simulink model "relative_distance_tracking4"  (R2018b)
settings: Solver=FixedStepAuto  StartTime=0.0  StopTime=15  FixedStep=dt  RelTol=1e-3
values from neighbouring files (symbols this model uses):
  C = [0 1]    [relative_distance_design4.m]
  CA = C*A    [relative_distance_design4.m]
  d0_ego = 0    [relative_distance_design4.m]
  d0_other = d0_ego + safe_dist0    (= 98.5)    [relative_distance_design4.m]
  fc = 0.5    [relative_distance_design4.m]
  fps2mph = 1/mph2fps    (= 0.680272108844)    [relative_distance_design4.m]
  g = 32.2    [relative_distance_design4.m]    (also in run_decel.m)
  invCB = inv(C*B)    [relative_distance_design4.m]
  Ka = 8    [relative_distance_design4.m]
  Kd = 0.25    [relative_distance_design4.m]
  Kdi = w_des^2    (= 4)    [relative_distance_design4.m]
  Kdp = 2*z_des*w_des    (= 4)    [relative_distance_design4.m]
  Kv = 2    [relative_distance_design4.m]
  max_accel = 0.6*g    (= 19.32)    [relative_distance_design4.m]
  min_accel = -1.0*g    (= -32.2)    [relative_distance_design4.m]
  mph2fps = 1.47    [relative_distance_design4.m]
  safe_dist0 = d0 + slope*(v0_ego*fps2mph)^2 + safe_dist0_margin    (= 98.5)    [relative_distance_design4.m]
  safe_dist_out = d0 + slope*v_in.^2 + safe_dist0_margin    [relative_distance_design4.m]
  v0_ego = 70*mph2fps    (= 102.9)    [relative_distance_design4.m]
  v0_other = v0_ego    (= 102.9)    [relative_distance_design4.m]
  v_in = (0:0.1:100)    [relative_distance_design4.m]
  v_other = v0_other + del_v0    (= 0)    [relative_distance_design4.m]
  wa_ego = 4    [relative_distance_design4.m]
settings Model: Creator=suvo.ganguli  LastModifiedBy=suvo.ganguli

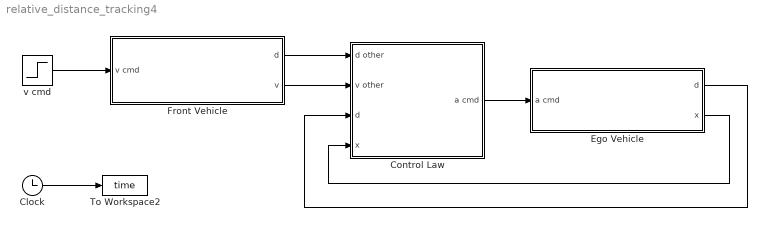
== system relative_distance_tracking4 ==
  Clock : Clock
  Control Law : Subsystem
  Ego Vehicle : Subsystem
  Front Vehicle : Subsystem
  To Workspace2 : ToWorkspace  VariableName=time  SampleTime=-1
  "v cmd " : Step  Before=v0_other  After=v_other  SampleTime=0
  wires:
  Clock/1 -> To Workspace2/1
  Control Law/1(a cmd) -> Ego Vehicle/1(a cmd)
  Ego Vehicle/2(x) -> Control Law/4(x)
  "v cmd "/1 -> Front Vehicle/1(v cmd)
  Ego Vehicle/1(d) -> Control Law/3(d)
  Front Vehicle/1(d) -> Control Law/1(d other)
  Front Vehicle/2(v) -> Control Law/2(v other)

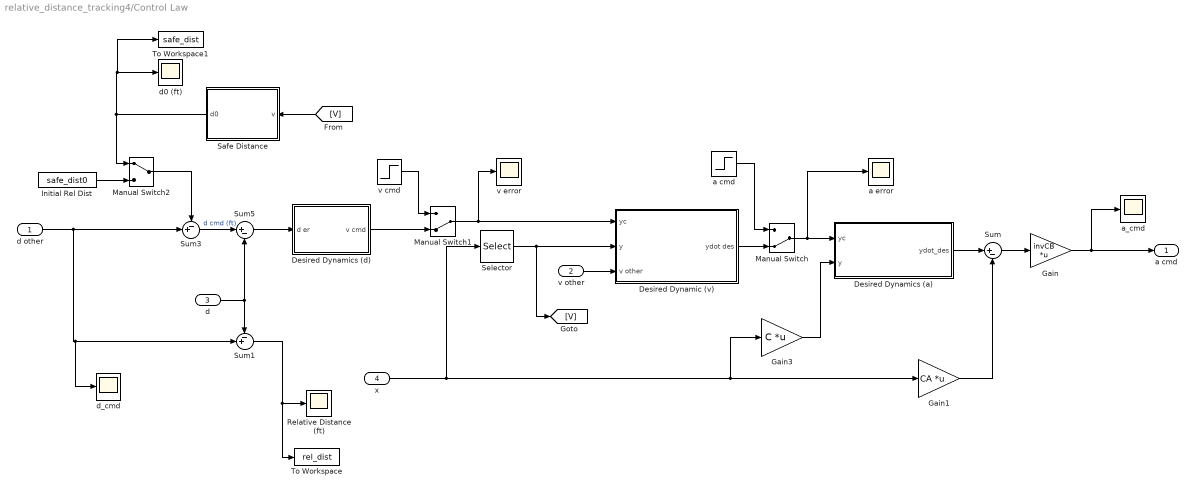
== system relative_distance_tracking4/Control Law ==
  d other : Inport
  v other : Inport  Port=2
  d : Inport  Port=3
  x : Inport  Port=4
  Desired Dynamic (v) : Subsystem
  Desired Dynamics (a) : Subsystem
  Desired Dynamics (d) : Subsystem
  Gain : Gain  Gain=invCB  Multiplication=Matrix(K*u)
  Gain1 : Gain  Gain=CA  Multiplication=Matrix(K*u)
  Gain3 : Gain  Gain=C  Multiplication=Matrix(K*u)
  Initial Rel Dist : Constant  Value=safe_dist0
  Manual Switch : ManualSwitch  CurrentSetting=0
  Manual Switch1 : ManualSwitch  CurrentSetting=0
  Manual Switch2 : ManualSwitch
  Relative Distance (ft) : Scope
  Safe Distance : Subsystem
  Selector : Selector  InputPortWidth=2  IndexOptions=Index vector (dialog)  Indices=1  OutputSizes=1
  Sum : Sum  Inputs=|+-
  Sum1 : Sum  Inputs=-+|
  Sum3 : Sum  Inputs=-+|
  Sum5 : Sum  Inputs=|+-
  To Workspace : ToWorkspace  VariableName=rel_dist  SampleTime=-1
  To Workspace1 : ToWorkspace  VariableName=safe_dist  SampleTime=-1
  "a cmd " : Step  After=0.6*32.2  SampleTime=0
  a error : Scope
  a_cmd : Scope
  d0 (ft) : Scope
  d_cmd : Scope
  v cmd : Step  After=10*mph2fps  SampleTime=0
  v error : Scope
  a cmd : Outport
  wires:
  x/1 -> Selector/1, Gain3/1, Gain1/1
  Gain1/1 -> Sum/2
  Gain/1 -> a_cmd/1, a cmd/1
  d other/1 -> d_cmd/1, Sum1/2, Sum3/2
  "a cmd "/1 -> Manual Switch/1
  Sum/1 -> Gain/1
  Manual Switch1/1 -> Desired Dynamic (v)/1(yc), v error/1
  v cmd/1 -> Manual Switch1/1
  Sum3/1 -> Sum5/1  "d cmd (ft)"
  d/1 -> Sum5/2, Sum1/1
  Sum1/1 -> Relative Distance (ft)/1, To Workspace/1
  Manual Switch/1 -> a error/1, Desired Dynamics (a)/1(yc)
  Desired Dynamics (a)/1(ydot_des) -> Sum/1
  Gain3/1 -> Desired Dynamics (a)/2(y)
  Sum5/1 -> Desired Dynamics (d)/1(d er)
  Desired Dynamics (d)/1(v cmd) -> Manual Switch1/2
  Initial Rel Dist/1 -> Manual Switch2/2
  Manual Switch2/1 -> Sum3/1
  [V] -> Safe Distance/1(v)
  Safe Distance/1(d0) -> Manual Switch2/1, To Workspace1/1, d0 (ft)/1
  Desired Dynamic (v)/1(ydot des) -> Manual Switch/2
  Selector/1 -> [V], Desired Dynamic (v)/2("y ")
  v other/1 -> Desired Dynamic (v)/3(v other)

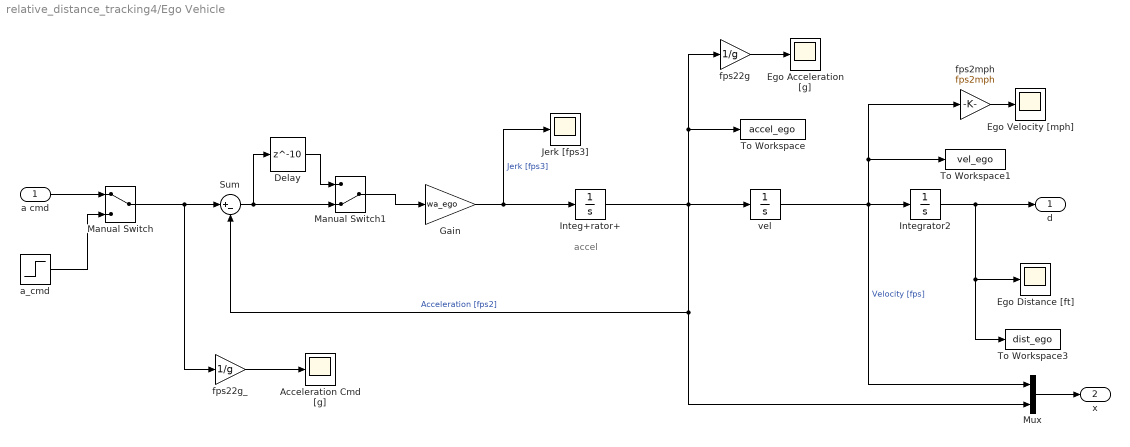
== system relative_distance_tracking4/Ego Vehicle ==
  note: accel
  a cmd : Inport
  Acceleration Cmd [g] : Scope
  Delay : Delay  DelayLength=10
  Ego Acceleration [g] : Scope
  Ego Distance [ft] : Scope
  Ego Velocity [mph] : Scope
  Gain : Gain  Gain=wa_ego
  Integ+rator+ : Integrator  LimitOutput=on  UpperSaturationLimit=max_accel  LowerSaturationLimit=min_accel
  Integrator2 : Integrator  InitialCondition=d0_ego
  Jerk [fps3] : Scope
  Manual Switch : ManualSwitch
  Manual Switch1 : ManualSwitch  CurrentSetting=0
  Mux : Mux  Inputs=2
  Sum : Sum  Inputs=|+-
  To Workspace : ToWorkspace  VariableName=accel_ego  SampleTime=-1
  To Workspace1 : ToWorkspace  VariableName=vel_ego  SampleTime=-1
  To Workspace3 : ToWorkspace  VariableName=dist_ego  SampleTime=-1
  a_cmd : Step  SampleTime=0
  fps22g : Gain  Gain=1/g
  fps22g_ : Gain  Gain=1/g
  fps2mph : Gain  Gain=fps2mph
  vel : Integrator  InitialCondition=v0_ego
  d : Outport
  x : Outport  Port=2
  wires:
  Gain/1 -> Jerk [fps3]/1, Integ+rator+/1  "Jerk [fps3]"
  fps2mph/1 -> Ego Velocity [mph]/1
  vel/1 -> Mux/1, Integrator2/1, To Workspace1/1, fps2mph/1  "Velocity [fps]"
  Integ+rator+/1 -> vel/1, To Workspace/1, fps22g/1, Mux/2, Sum/2  "Acceleration [fps2]"
  Integrator2/1 -> Ego Distance [ft]/1, To Workspace3/1, d/1
  fps22g/1 -> Ego Acceleration [g]/1
  Manual Switch/1 -> fps22g_/1, Sum/1
  a_cmd/1 -> Manual Switch/2
  a cmd/1 -> Manual Switch/1
  Mux/1 -> x/1
  fps22g_/1 -> Acceleration Cmd [g]/1
  Manual Switch1/1 -> Gain/1
  Sum/1 -> Delay/1, Manual Switch1/2
  Delay/1 -> Manual Switch1/1

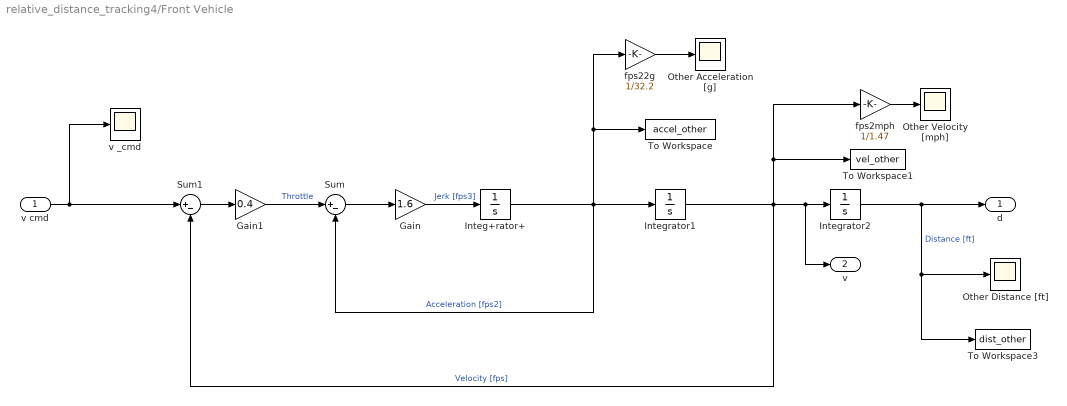
== system relative_distance_tracking4/Front Vehicle ==
  v cmd : Inport
  Gain : Gain  Gain=1.6
  Gain1 : Gain  Gain=0.4
  Integ+rator+ : Integrator  LimitOutput=on  UpperSaturationLimit=max_accel  LowerSaturationLimit=min_accel
  Integrator1 : Integrator  InitialCondition=v0_other
  Integrator2 : Integrator  InitialCondition=d0_other
  Other Acceleration [g] : Scope
  Other Distance [ft] : Scope
  Other Velocity [mph] : Scope
  Sum : Sum  Inputs=|+-
  Sum1 : Sum  Inputs=|+-
  To Workspace : ToWorkspace  VariableName=accel_other  SampleTime=-1
  To Workspace1 : ToWorkspace  VariableName=vel_other  SampleTime=-1
  To Workspace3 : ToWorkspace  VariableName=dist_other  SampleTime=-1
  fps22g : Gain  Gain=1/32.2
  fps2mph : Gain  Gain=1/1.47
  v _cmd : Scope
  d : Outport
  v : Outport  Port=2
  wires:
  Gain1/1 -> Sum/1  "Throttle"
  v cmd/1 -> Sum1/1, v _cmd/1
  fps22g/1 -> Other Acceleration [g]/1
  Sum1/1 -> Gain1/1
  Integ+rator+/1 -> Sum/2, fps22g/1, To Workspace/1, Integrator1/1  "Acceleration [fps2]"
  Sum/1 -> Gain/1
  Integrator1/1 -> fps2mph/1, To Workspace1/1, v/1, Integrator2/1, Sum1/2  "Velocity [fps]"
  fps2mph/1 -> Other Velocity [mph]/1
  Gain/1 -> Integ+rator+/1  "Jerk [fps3]"
  Integrator2/1 -> d/1, To Workspace3/1, Other Distance [ft]/1  "Distance [ft]"

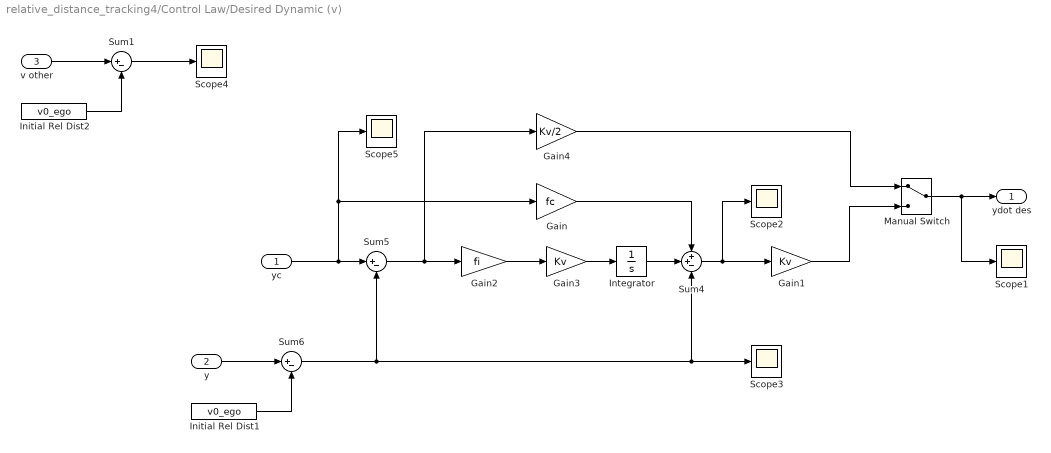
== system relative_distance_tracking4/Control Law/Desired Dynamic (v) ==
  yc : Inport
  "y " : Inport  Port=2
  v other : Inport  Port=3
  Gain : Gain  Gain=fc
  Gain1 : Gain  Gain=Kv
  Gain2 : Gain  Gain=fi
  Gain3 : Gain  Gain=Kv
  Gain4 : Gain  Gain=Kv/2
  Initial Rel Dist1 : Constant  Value=v0_ego
  Initial Rel Dist2 : Constant  Value=v0_ego
  Integrator : Integrator
  Manual Switch : ManualSwitch
  Scope{1..5} (5 alike) : Scope
  Sum1 : Sum  Inputs=|+-
  Sum4 : Sum  Inputs=++-
  Sum5 : Sum  Inputs=|+-
  Sum6 : Sum  Inputs=|+-
  ydot des : Outport
  wires:
  "y "/1 -> Sum6/1
  Initial Rel Dist1/1 -> Sum6/2
  Gain3/1 -> Integrator/1
  Gain/1 -> Sum4/1
  Gain2/1 -> Gain3/1
  Sum5/1 -> Gain4/1, Gain2/1
  Sum4/1 -> Gain1/1, Scope2/1
  Integrator/1 -> Sum4/2
  Manual Switch/1 -> Scope1/1, ydot des/1
  Gain4/1 -> Manual Switch/1
  Sum6/1 -> Scope3/1, Sum4/3, Sum5/2
  Gain1/1 -> Manual Switch/2
  yc/1 -> Gain/1, Scope5/1, Sum5/1
  v other/1 -> Sum1/1
  Initial Rel Dist2/1 -> Sum1/2
  Sum1/1 -> Scope4/1

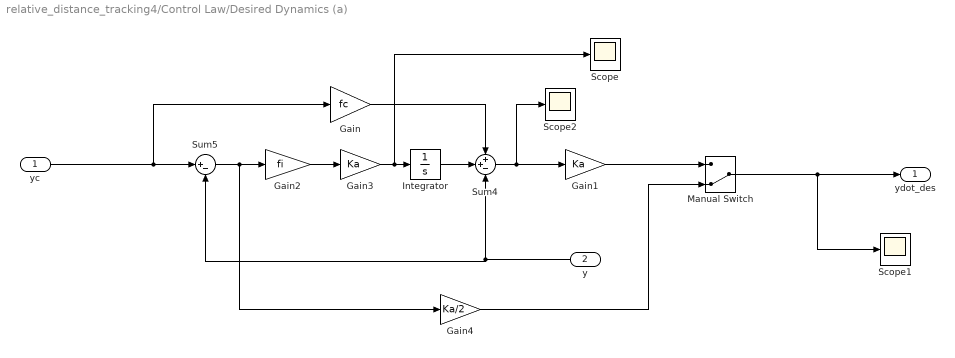
== system relative_distance_tracking4/Control Law/Desired Dynamics (a) ==
  yc : Inport
  y : Inport  Port=2
  Gain : Gain  Gain=fc
  Gain1 : Gain  Gain=Ka
  Gain2 : Gain  Gain=fi
  Gain3 : Gain  Gain=Ka
  Gain4 : Gain  Gain=Ka/2
  Integrator : Integrator
  Manual Switch : ManualSwitch  CurrentSetting=0
  Scope : Scope
  Scope1 : Scope
  Scope2 : Scope
  Sum4 : Sum  Inputs=++-
  Sum5 : Sum  Inputs=|+-
  ydot_des : Outport
  wires:
  Gain4/1 -> Manual Switch/2
  Manual Switch/1 -> ydot_des/1, Scope1/1
  Gain1/1 -> Manual Switch/1
  Gain3/1 -> Integrator/1, Scope/1
  y/1 -> Sum4/3, Sum5/2
  Gain/1 -> Sum4/1
  Integrator/1 -> Sum4/2
  yc/1 -> Sum5/1, Gain/1
  Sum5/1 -> Gain2/1, Gain4/1
  Gain2/1 -> Gain3/1
  Sum4/1 -> Gain1/1, Scope2/1

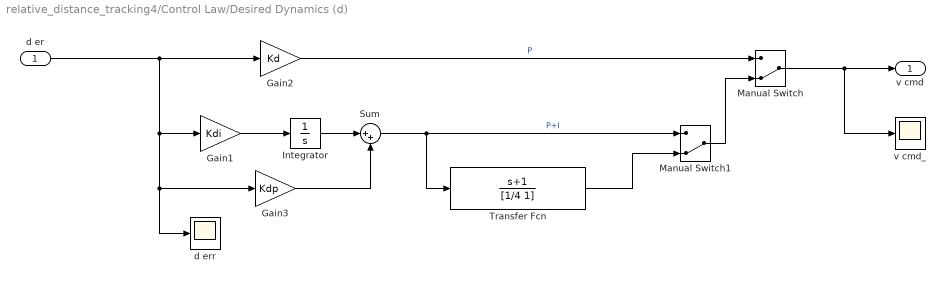
== system relative_distance_tracking4/Control Law/Desired Dynamics (d) ==
  d er : Inport
  Gain1 : Gain  Gain=Kdi
  Gain2 : Gain  Gain=Kd
  Gain3 : Gain  Gain=Kdp
  Integrator : Integrator
  Manual Switch : ManualSwitch  CurrentSetting=0
  Manual Switch1 : ManualSwitch  CurrentSetting=0
  Sum : Sum  Inputs=|++
  Transfer Fcn : TransferFcn  Numerator=[1 1]  Denominator=[1/4 1]
  "d err " : Scope
  v cmd_ : Scope
  v cmd : Outport
  wires:
  Gain2/1 -> Manual Switch/1  "P"
  Manual Switch/1 -> v cmd_/1, v cmd/1
  Gain1/1 -> Integrator/1
  Integrator/1 -> Sum/1
  Gain3/1 -> Sum/2
  Manual Switch1/1 -> Manual Switch/2
  Sum/1 -> Transfer Fcn/1, Manual Switch1/1  "P+I"
  Transfer Fcn/1 -> Manual Switch1/2
  d er/1 -> "d err "/1, Gain3/1, Gain1/1, Gain2/1

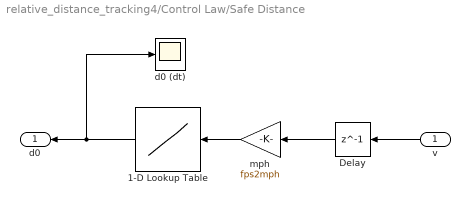
== system relative_distance_tracking4/Control Law/Safe Distance ==
  v : Inport
  1-D Lookup Table : Lookup_n-D  NumberOfTableDimensions=1  BreakpointsForDimension1=v_in  Table=safe_dist_out  InternalRulePriority=Speed  RndMeth=Simplest  InputSameDT=on
  Delay : Delay  DelayLength=1  InitialCondition=v0_ego
  d0 (dt) : Scope
  mph : Gain  Gain=fps2mph
  d0 : Outport
  wires:
  mph/1 -> 1-D Lookup Table/1
  v/1 -> Delay/1
  1-D Lookup Table/1 -> d0 (dt)/1, d0/1
  Delay/1 -> mph/1
